simulink model "EHB_speedgoat_R2020a_V1"  (R2020a)
settings: Solver=FixedStepDiscrete  StartTime=0.0  StopTime=inf  FixedStep=0.001  RelTol=1e-3  EnableMultiTasking=on
model workspace (MAT data in the model file):
  A = Simulink.Signal
  A.DataType = 'uint8'
  A.Dimensions = 13
  A.DimensionsMode = 'auto'
  A.Complexity = 'auto'
  A.SampleTime = -1
  A.SamplingMode = 'auto'
  B = Simulink.Signal
  B.DataType = 'uint8'
  B.Dimensions = 13
  B.DimensionsMode = 'auto'
  B.Complexity = 'auto'
  B.SampleTime = -1
  B.SamplingMode = 'auto'
  C = Simulink.Signal
  C.DataType = 'uint8'
  C.Dimensions = 13
  C.DimensionsMode = 'auto'
  C.Complexity = 'auto'
  C.SampleTime = -1
  C.SamplingMode = 'auto'
  D = Simulink.Signal
  D.DataType = 'uint8'
  D.Dimensions = 13
  D.DimensionsMode = 'auto'
  D.Complexity = 'auto'
  D.SampleTime = -1
  D.SamplingMode = 'auto'
  E = Simulink.Signal
  E.DataType = 'uint8'
  E.Dimensions = 13
  E.DimensionsMode = 'auto'
  E.Complexity = 'auto'
  E.SampleTime = -1
  E.SamplingMode = 'auto'
  calin = [-9.96 -7.98 -5.98 -3.99 -1.994 0 1.995 3.992 5.99 7.98 9.97]
  calout = [-10 -8 -6 -4 -2 0 2 4 6 8 10]
undefined symbols (not defined in the file): Com1, none, ts_IO612
libraries: simulink x1436, xpcethercatlib x1223, yisutbxlib_utilities x256, xpcutilitieslib x156, hdlsllib x145, canmsglib x46, speedgoatlib_IO602_4 x11, speedgoatlib_IO611 x7, slrttcplib x4, CanManageLib x3, slrtlib x3, xpcseriallib x2
(part 1 of 30)
settings Model: xpc_rtwmakecfg_data=_xpcethercatlib_  SimulationMode=external  Creator=xiaoming  LastModifiedBy=17802
settings SolverCC: ConcurrentTasks=on  AutoInsertRateTranBlk=on
settings DataIOCC: SaveFormat=StructureWithTime  SaveState=on  SignalLoggingName=logsOut
settings OptimizationCC: BlockReduction=off  BooleanDataType=off  OptimizeBlockIOStorage=off  BufferReuse=off  GlobalBufferReuse=off  ExpressionFolding=off  LocalBlockOutputs=off  InitFltsAndDblsToZero=on  OptimizeDataStoreBuffers=off  BusAssignmentInplaceUpdate=off
settings DebuggingCC: SaveWithParameterizedLinksMsg=none  UnderspecifiedInitializationDetection=Classic  MergeDetectMultiDrivingBlocksExec=none  CheckExecutionContextPreStartOutputMsg=on  CheckExecutionContextRuntimeOutputMsg=on  SignalResolutionControl=TryResolveAllWithWarning  SFUnexpectedBacktrackingDiag=warning  SFNoUnconditionalDefaultTransitionDiag=warning  SFExecutionAtInitializationDiag=none  ArithmeticOperatorsInVariantConditions=warning
settings HardwareCC: ProdBitPerPointer=32  ProdBitPerSizeT=32  ProdBitPerPtrDiffT=32  ProdLargestAtomicFloat=None  ProdWordSize=32  ProdLongLongMode=on  ProdHWDeviceType=Generic->32-bit x86 compatible
settings ModelReferenceCC: PropagateSignalLabelsOutOfModel=off
settings SFSimCC: SimUseLocalCustomCode=off
settings RTWCC: Description=Simulink Real-Time  SystemTargetFile=slrt.tlc  TemplateMakefile=slrt_default_tmf  RTWUseLocalCustomCode=off  CodeExecutionProfiling=on  RTWCompilerOptimization=on
settings CodeAppCC: StateflowObjectComments=on
settings SimulinkRealTimeCC: SupportVariableSizeSignals=on  RL32LogTETModifier=off  xPCConcurrentTasks=on
settings ConfigComp: CovMetricSettings=dw  CovHtmlReporting=on  CovSaveCumulativeToWorkspaceVar=on  CovSaveSingleToWorkspaceVar=on  CovExternalEMLEnable=off  CovSFcnEnable=off

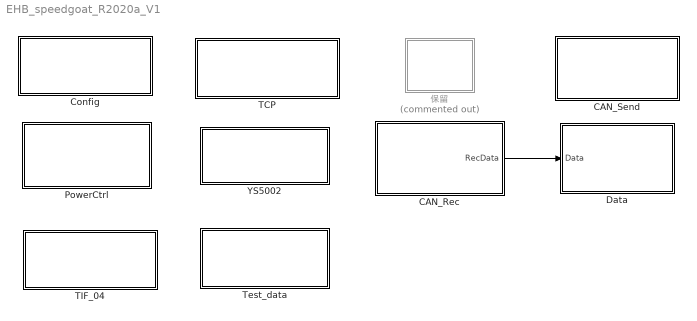
== system EHB_speedgoat_R2020a_V1 ==
  CAN_Rec : Subsystem
  CAN_Send : Subsystem
  Config : Subsystem
  Data : Subsystem
  PowerCtrl : Subsystem
  TCP : Subsystem
  TIF_04 : Subsystem
  Test_data : Subsystem
  YS5002 : Subsystem
  保留 : Subsystem  Commented=on
  wires:
  CAN_Rec/1(RecData) -> Data/1(Data)

== system EHB_speedgoat_R2020a_V1/CAN_Rec ==
  CAN Receive : Subsystem  TreatAsAtomicUnit=on
  RecData : Outport
  wires:
  CAN Receive/1(RecData) -> RecData/1

== system EHB_speedgoat_R2020a_V1/CAN_Send ==
  Bus Creator : BusCreator  Inputs=2
  CAN Transmit : Subsystem  TreatAsAtomicUnit=on
  Enable : BusSelector  OutputSignals=Trigger.Enable_CanTransmit
  Signal : Subsystem
  Trigger : Subsystem
  wires:
  Trigger/1(Trigger) -> Bus Creator/1  "Trigger"
  Signal/1(Signal) -> Bus Creator/2  "Signal"
  Bus Creator/1 -> CAN Transmit/1(Data), Enable/1  "Data"
  Enable/1 -> CAN Transmit/Enable  "<Enable_CanTransmit>"

== system EHB_speedgoat_R2020a_V1/Config ==
  CAN & LIN Setup : speedgoatlib_IO611/Legacy/CAN & LIN Setup  Commented=on  id=1  drvLtr=C:  PCISlot=-1  port1=CAN (HS/LS)  port2=CAN (HS/LS)  port3=LIN  port4=LIN  opModeCAN1=Highspeed (HS)  bdrCAN1=1 MBaud  usrBdrCAN1=[5, 1, 13, 2]  bdrFD1=5 MBaud  usrBdrFD1=[2, 1, 5, 2, 75, 5000]  stdAccMaskCAN1=[0, 0]  extAccMaskCAN1=[0, 0]  opModeCAN2=Highspeed (HS)  bdrCAN2=1 MBaud  usrBdrCAN2=[5, 1, 13, 2]  bdrFD2=5 MBaud  usrBdrFD2=[2, 1, 5, 2, 75, 5000]  stdAccMaskCAN2=[0, 0]  extAccMaskCAN2=[0, 0]  initStruct=[]  termStruct=[]  opModeLIN3=Master  bdrLIN3=19200  opModeLIN4=Slave  bdrLIN4=19200  protl=IO611  qtyMod=1  chNo=[1, 2, 3, 4]  ptTypes=[1, 1, 2, 2]  isProtlFD=[0, 0]  protlHelpIdx=[0, 1, 0, 1]  isFDMod=1
      settings: SourceProductName=Simulink Real-Time: Speedgoat I/O Blockset
  "CAN Setup " : speedgoatlib_IO602_4/Legacy/CAN Setup   moduletype=IO602  id=1  pciSlot=-1  chn1=CAN (HS)  chn2=CAN (HS)  chn3=CAN (HS)  chn4=CAN (HS)  initStruct=[]  termStruct=[]  ArbitrationbdrChn1=500 kBaud  ArbitrationManbdrChn1=[2,16,63,16]  FdbdrChn1=5.0 MBaud  FdManbdrChn1=[2,2,5,2]  ArbitrationbdrChn2=500 kBaud  ArbitrationManbdrChn2=[2,16,63,16]  FdbdrChn2=5.0 MBaud  FdManbdrChn2=[2,2,5,2]  ArbitrationbdrChn3=500 kBaud  ArbitrationManbdrChn3=[2,16,63,16]  FdbdrChn3=5.0 MBaud  FdManbdrChn3=[2,2,5,2]  ArbitrationbdrChn4=500 kBaud  ArbitrationManbdrChn4=[2,16,63,16]  FdbdrChn4=5.0 MBaud  FdManbdrChn4=[2,2,5,2]  moduleInitValues=[602 1 -1 -1]
      settings: SourceProductName=Simulink Real-Time: Speedgoat I/O Blockset
  Constant : Constant
  Gain{,1..5} (6 alike) : Gain
  HILReady : simulink/Logic and Bit Operations/Compare To Constant  relop===  const=8  OutDataTypeStr=boolean
  Selector : Selector  InputPortWidth=6  IndexOptions=Index vector (dialog)  Indices=[2]  OutputSizes=1
  TCP Client Configure : Subsystem  Priority=-1  AncestorBlock=slrttcplib/TCP Client Configure  InitFcn=|  TreatAsAtomicUnit=on  mask(slrttcpclientconfig){useHostTargetConn=off, clientAddress=192.168.0.55, clientPort=25001, SubnetMask=255.255.255.0, Gateway=0.0.0.0, remoteAddress=192.168.0.178, remotePort=4001, PciBus=[6], PciSlot=[0], PciFunction=[0]}
      | % Validate model
      | tcpvalidatemodel(gcb);
      mask prompts: useHostTargetConn "Use host-target connection"; clientAddress "Client IP address:"; clientPort "Client local port:"; SubnetMask "Subnet mask:"; remoteAddress "Remote server IP address:"; remotePort "Remote server port:"; PciBus "PCI Bus:"; PciSlot "Slot:"; PciFunction "Function:"
      mask help: Configure a TCP client application that uses the specified Ethernet interface.
      mask init:
      | % Validate mask parameter values
      | tcpslgate('privateTCPClientConfig', gcb, 'validateParams', clientAddress, clientPort, remoteAddress, remotePort, SubnetMask, Gateway, PciBus, PciSlot, PciFunction);
      mask Help: eval('xpcdoc(''TCP_ClientConfig'')');
      mask TypeOptions useHostTargetConn: TCP Client/useHostTargetConn | IP Configure/disable
      mask Callback useHostTargetConn: tcpslgate('privateTCPClientConfig', gcb, 'toggleMaskVisible');
      mask TypeOptions clientAddress: IP Configure/IpAddress | TCP Client/clientAddress
      mask TypeOptions clientPort: TCP Client/clientPort
      mask TypeOptions SubnetMask: IP Configure/SubnetMask
      mask TypeOptions Gateway: IP Configure/Gateway
      mask TypeOptions remoteAddress: TCP Client/remoteAddress
      mask TypeOptions remotePort: TCP Client/remotePort
      mask TypeOptions PciBus: IP Configure/PciBus
      mask TypeOptions PciSlot: IP Configure/PciSlot
      mask TypeOptions PciFunction: IP Configure/PciFunction
      mask DialogControl DescGroupVar Prompt: Configure TCP Client
      mask Display:
      | maskDisplay = tcpslgate('privateTCPClientConfig', gcb, 'dispStr', clientAddress, clientPort, remoteAddress, remotePort, SubnetMask, Gateway, PciBus, PciSlot, PciFunction);
      | disp(maskDisplay);
      | 
      | port_label('input', 1, 'Enable')
      | port_label('output', 1, 'Status')
  Terminator{,1..5} (6 alike) : Terminator
  YISU Toolbox Init : Subsystem  mask(ystbx_init){eniFile=D:\Matlab\EHB_Prj\data\ENI\HuDa.xml, deviceIdx=0, pciBus=7, pciSlot=0, pciFcn=0, outStatusInfo=on}
      mask prompts: eniFile "Config File(ENI):"; deviceIdx "Device Index:"; pciBus "PCI Bus:"; pciSlot "PCI Slot:"; pciFcn "PCI Function:"; outStatusInfo "Enable Status Info Output"
      mask help: 基于EtherCat Init模块，配置ENI文件并设定设备ID等信息
      mask DialogControl selectFile Prompt: Browse
      mask DialogControl selectFile Callback: ystbx.mask.callbacks.init_selectFile();
      mask DialogControl applyButton Prompt: Apply Modification
      mask DialogControl applyButton Callback: ystbx.mask.callbacks.maskApply();
      mask Display: disp('YISU Toolbox Init\nNetwork Device 0');port_label('output', 1, 'Status');
  wires:
  HILReady/1 -> Gain/1
  Selector/1 -> HILReady/1
  Constant/1 -> TCP Client Configure/5(In5), TCP Client Configure/4(In4), TCP Client Configure/3(In3), TCP Client Configure/2(In2), TCP Client Configure/1(In1)
  TCP Client Configure/1(Out1) -> Gain1/1
  TCP Client Configure/2(Out2) -> Gain2/1
  TCP Client Configure/3(Out3) -> Gain3/1
  TCP Client Configure/4(Out4) -> Gain4/1
  TCP Client Configure/5(Out5) -> Gain5/1
  YISU Toolbox Init/1(Status) -> Selector/1
  Gain/1 -> Terminator/1
  Gain1/1 -> Terminator1/1
  Gain2/1 -> Terminator2/1
  Gain3/1 -> Terminator3/1
  Gain4/1 -> Terminator4/1
  Gain5/1 -> Terminator5/1

== system EHB_speedgoat_R2020a_V1/Data ==
  note: EHB工作状态
  note: 制动状态反馈
  note: EHB故障等级
  note: 当前实际制动液压力
  note: 制动指令异常
  note: EHB液压力跟随轻微异常
  note: EHB液压力轻微震荡
  note: 温度传感器部分故障
  note: 温度传感器完全故障
  note: 液压力传感器故障
  note: 控制器温度过高
  note: 供电电压过低异常
  note: 供电电压过高异常
  note: EHB液压力跟随严重异常
  note: EHB液压力严重震荡
  note: 负载失配故障
  note: CAN通信故障
  note: EHB过流故障
  note: 电流传感器故障
  note: 供电电压过低故障
  note: 供电电压过高故障
  note: 功率开关故障
  note: 预驱故障
  note: EHB电机位置失效
  note: EHB软件版本号
  note: EHB硬件版本号
  note: 左前轮轮速
  note: 左前轮轮速有效性
  note: 右前轮轮速
  note: 右前轮轮速有效性
  note: 左后轮轮速
  note: 左后轮轮速有效性
  note: 右后轮轮速
  note: 右后轮轮速有效性
  Data : Inport
  Bus Selector : BusSelector  OutputSignals=CAN_Msg_0x125.EHB_Status,CAN_Msg_0x125.EHB_BrakeCondition,CAN_Msg_0x125.EHB_EHBFaultLevel,CAN_Msg_0x125.EHB_ActualPressure
  Bus Selector1 : BusSelector  OutputSignals=CAN_Msg_0x126.EHB_BrkReqWarn,CAN_Msg_0x126.EHB_PFolwFltLv1,CAN_Msg_0x126.EHB_PCtrlVibLv1,CAN_Msg_0x126.EHB_NTCFltLv1,CAN_Msg_0x126.EHB_NTCFltLv2,CAN_Msg_0x126.EHB_PSnsrFlt,CAN_Msg_0x126.EHB_OverTempWarn,CAN_Msg_0x126.EHB_USplyLowLv1,CAN_Msg_0x126.EHB_USplyHighLv1,CAN_Msg_0x126.EHB_PFolwFltLv2,CAN_Msg_0x126.EHB_PCtrlVibLv2,CAN_Msg_0x126.EHB_LoadMismatchFlt,CAN_Msg_0x126.EHB_CANBusOff,CAN_Msg_0x126.EHB_OverIFlt,CAN_Msg_0x126.EHB_ISnsrFlt,CAN_Msg_0x126.EHB_USplyLowLv2,CAN_Msg_0x126.EHB_USplyHighLv2,CAN_Msg_0x126.EHB_PwrSwtFlt,CAN_Msg_0x126.EHB_PwrDrvrFlt,CAN_Msg_0x126.EHB_MotPosnFlt,CAN_Msg_0x126.EHB_SoftwareVersion,CAN_Msg_0x126.EHB_HardwareVersion
  Bus Selector2 : BusSelector  OutputSignals=CAN_Msg_0x127.EHB_WhlFLSpd,CAN_Msg_0x127.EHB_WhlFLSpdVld,CAN_Msg_0x127.EHB_WhlFRSpd,CAN_Msg_0x127.EHB_WhlFRSpdVld,CAN_Msg_0x127.EHB_WhlRLSpd,CAN_Msg_0x127.EHB_WhlRLSpdVld,CAN_Msg_0x127.EHB_WhlRRSpd,CAN_Msg_0x127.EHB_WhlRRSpdVld
  Bus Selector3 : BusSelector  OutputSignals=Message_1_0x281.U_Current,Message_1_0x281.V_Current,Message_1_0x281.W_Current,Message_1_0x281.Angle1
  Bus Selector4 : BusSelector  OutputSignals=Message_3_0x283.ia_act,Message_3_0x283.ib_act
  Gain{,1..39} (40 alike) : Gain
  Terminator{,1..39} (40 alike) : Terminator
  wires:
  Data/1 -> Bus Selector3/1, Bus Selector2/1, [Data], Bus Selector1/1, Bus Selector/1
  Gain/1 -> Terminator/1
  Bus Selector/1 -> Gain/1  "<EHB_Status>"
  Gain1/1 -> Terminator1/1
  Bus Selector/2 -> Gain1/1  "<EHB_BrakeCondition>"
  Gain2/1 -> Terminator2/1
  Bus Selector/3 -> Gain2/1  "<EHB_EHBFaultLevel>"
  Gain3/1 -> Terminator3/1
  Bus Selector/4 -> Gain3/1  "<EHB_ActualPressure>"
  Gain7/1 -> Terminator7/1
  Gain6/1 -> Terminator6/1
  Gain5/1 -> Terminator5/1
  Gain4/1 -> Terminator4/1
  Bus Selector1/1 -> Gain4/1  "<EHB_BrkReqWarn>"
  Bus Selector1/2 -> Gain5/1  "<EHB_PFolwFltLv1>"
  Bus Selector1/3 -> Gain6/1  "<EHB_PCtrlVibLv1>"
  Bus Selector1/4 -> Gain7/1  "<EHB_NTCFltLv1>"
  Gain8/1 -> Terminator8/1
  Gain9/1 -> Terminator9/1
  Gain10/1 -> Terminator10/1
  Gain11/1 -> Terminator11/1
  Gain13/1 -> Terminator13/1
  Gain12/1 -> Terminator12/1
  Gain19/1 -> Terminator19/1
  Gain18/1 -> Terminator18/1
  Gain14/1 -> Terminator14/1
  Gain15/1 -> Terminator15/1
  Gain16/1 -> Terminator16/1
  Gain17/1 -> Terminator17/1
  Gain25/1 -> Terminator25/1
  Gain24/1 -> Terminator24/1
  Gain23/1 -> Terminator23/1
  Gain22/1 -> Terminator22/1
  Gain26/1 -> Terminator26/1
  Gain27/1 -> Terminator27/1
  Bus Selector1/5 -> Gain8/1  "<EHB_NTCFltLv2>"
  Bus Selector1/6 -> Gain9/1  "<EHB_PSnsrFlt>"
  Bus Selector1/7 -> Gain10/1  "<EHB_OverTempWarn>"
  Bus Selector1/8 -> Gain11/1  "<EHB_USplyLowLv1>"
  Bus Selector1/9 -> Gain14/1  "<EHB_USplyHighLv1>"
  Bus Selector1/10 -> Gain15/1  "<EHB_PFolwFltLv2>"
  Bus Selector1/11 -> Gain16/1  "<EHB_PCtrlVibLv2>"
  Bus Selector1/12 -> Gain17/1  "<EHB_LoadMismatchFlt>"
  Bus Selector1/13 -> Gain18/1  "<EHB_CANBusOff>"
  Bus Selector1/14 -> Gain19/1  "<EHB_OverIFlt>"
  Bus Selector1/15 -> Gain12/1  "<EHB_ISnsrFlt>"
  Bus Selector1/16 -> Gain13/1  "<EHB_USplyLowLv2>"
  Bus Selector1/17 -> Gain22/1  "<EHB_USplyHighLv2>"
  Bus Selector1/18 -> Gain23/1  "<EHB_PwrSwtFlt>"
  Bus Selector1/19 -> Gain24/1  "<EHB_PwrDrvrFlt>"
  Bus Selector1/20 -> Gain25/1  "<EHB_MotPosnFlt>"
  Bus Selector1/21 -> Gain26/1  "<EHB_SoftwareVersion>"
  Bus Selector1/22 -> Gain27/1  "<EHB_HardwareVersion>"
  Gain29/1 -> Terminator29/1
  Gain28/1 -> Terminator28/1
  Gain21/1 -> Terminator21/1
  Gain20/1 -> Terminator20/1
  Gain30/1 -> Terminator30/1
  Gain31/1 -> Terminator31/1
  Gain32/1 -> Terminator32/1
  Gain33/1 -> Terminator33/1
  Bus Selector2/1 -> Gain20/1  "<EHB_WhlFLSpd>"
  Bus Selector2/2 -> Gain21/1  "<EHB_WhlFLSpdVld>"
  Bus Selector2/3 -> Gain28/1  "<EHB_WhlFRSpd>"
  Bus Selector2/4 -> Gain29/1  "<EHB_WhlFRSpdVld>"
  Bus Selector2/5 -> Gain30/1  "<EHB_WhlRLSpd>"
  Bus Selector2/6 -> Gain31/1  "<EHB_WhlRLSpdVld>"
  Bus Selector2/7 -> Gain32/1  "<EHB_WhlRRSpd>"
  Bus Selector2/8 -> Gain33/1  "<EHB_WhlRRSpdVld>"
  Gain37/1 -> Terminator37/1
  Gain36/1 -> Terminator36/1
  Gain35/1 -> Terminator35/1
  Gain34/1 -> Terminator34/1
  Bus Selector3/1 -> Gain34/1  "<U_Current>"
  Bus Selector3/2 -> Gain35/1  "<V_Current>"
  Bus Selector3/3 -> Gain36/1  "<W_Current>"
  Bus Selector3/4 -> Gain37/1  "<Angle1>"
  [Data] -> Bus Selector4/1
  Gain38/1 -> Terminator38/1
  Gain39/1 -> Terminator39/1
  Bus Selector4/1 -> Gain38/1  "<ia_act>"
  Bus Selector4/2 -> Gain39/1  "<ib_act>"

== system EHB_speedgoat_R2020a_V1/PowerCtrl ==
  CurrSet[A] : Constant  OutDataTypeStr=uint16
  OnOff : Constant  OutDataTypeStr=uint8
  PowerCtrl : Subsystem
  PowerPosSet[W] : Constant  Value=6000  OutDataTypeStr=uint16
  Toggle Switch : ToggleSwitchBlock  LabelPosition=Hide
      settings: Values={{'Off', 'On'}, [0 1]}
  VoltValue[V] : Constant  Value=12  OutDataTypeStr=uint32
  wires:
  CurrSet[A]/1 -> PowerCtrl/3(CurrSet[A])  "CurrSet[A]"
  [Power_V] -> PowerCtrl/1(VoltValue[V])  "VoltValue[V]"
  OnOff/1 -> PowerCtrl/2(OnOff)  "OnOff"
  PowerPosSet[W]/1 -> PowerCtrl/4(PowerPosSet[W])  "PowerPosSet[W]"

== system EHB_speedgoat_R2020a_V1/TCP ==
  Constant{,1..3} (4 alike) : Constant
  Counter Limited1 : simulink/Sources/Counter Limited  uplimit=7  tsamp=0.1
  Counter Limited3 : simulink/Sources/Counter Limited  uplimit=6  tsamp=0.1
  From1 : From  Commented=on  GotoTag=YS4008_M_3  TagVisibility=global
  From11 : From  Commented=on  GotoTag=YS4008_M_2  TagVisibility=global
  From15 : From  Commented=on  GotoTag=YS7501_M  TagVisibility=global
  From18 : From  Commented=on  GotoTag=YS4008_M_4  TagVisibility=global
  From19 : From  Commented=on  GotoTag=YS4008_M_1  TagVisibility=global
  From20 : From  Commented=on  GotoTag=YS4008_M_5  TagVisibility=global
  From21 : From  Commented=on  GotoTag=YS4008_M_6  TagVisibility=global
  From22 : From  Commented=on  GotoTag=YS4020_M_2_1  TagVisibility=global
  From24 : From  Commented=on  GotoTag=YS4020_M_2_2  TagVisibility=global
  From6 : From  Commented=on  GotoTag=YS4020_M_1_2  TagVisibility=global
  From9 : From  Commented=on  GotoTag=YS4020_M_1_1  TagVisibility=global
  Ground{,1..10} (11 alike) : Ground
  Multiport Switch1 : MultiPortSwitch  DataPortOrder=Zero-based contiguous  Inputs=8  DiagnosticForDefault=None  zeroidx=on
  Multiport Switch2 : MultiPortSwitch  DataPortOrder=Zero-based contiguous  Inputs=7  DiagnosticForDefault=None  zeroidx=on
  TCP Send : slrttcplib/TCP Send  socketAddPortVal=Client: 192.168.0.55:25001  sampleTime=-1
      settings: SourceProductBaseCode=XP
  TCP Send1 : slrttcplib/TCP Send  socketAddPortVal=Client: 192.168.0.55:25002  sampleTime=-1
      settings: SourceProductBaseCode=XP
  TCP Send2 : slrttcplib/TCP Send  socketAddPortVal=Client: 192.168.0.55:25003  sampleTime=-1
      settings: SourceProductBaseCode=XP
  TCP Send3 : slrttcplib/TCP Send  socketAddPortVal=Client: 192.168.0.55:25004  sampleTime=-1
      settings: SourceProductBaseCode=XP
  Terminator{,1..3} (4 alike) : Terminator
  Width{,1..3} (4 alike) : Width
  wires:
  Width/1 -> TCP Send/3
  [PowerPosSet] -> Multiport Switch2/4
  [CurrSet] -> Multiport Switch2/3
  [VoltSet] -> Multiport Switch2/2
  Ground/1 -> Multiport Switch1/2
  Multiport Switch1/1 -> TCP Send/2, Width/1
  [YS5002] -> Multiport Switch2/5
  Ground8/1 -> Multiport Switch2/6
  Ground9/1 -> Multiport Switch2/7
  Ground4/1 -> Multiport Switch1/3
  Ground1/1 -> Multiport Switch1/4
  Ground5/1 -> Multiport Switch1/5
  [Enable] -> Width2/1, TCP Send2/2
  Ground6/1 -> Multiport Switch1/7
  Ground2/1 -> Multiport Switch1/6
  Ground10/1 -> Multiport Switch2/8
  Constant/1 -> TCP Send/1
  TCP Send/1 -> Terminator/1
  TCP Send1/1 -> Terminator1/1
  Constant1/1 -> TCP Send1/1
  Multiport Switch2/1 -> TCP Send1/2, Width1/1
  Width1/1 -> TCP Send1/3
  Constant2/1 -> TCP Send2/1
  Width2/1 -> TCP Send2/3
  TCP Send2/1 -> Terminator2/1
  Counter Limited1/1 -> Multiport Switch1/1
  Counter Limited3/1 -> Multiport Switch2/1
  TCP Send3/1 -> Terminator3/1
  Width3/1 -> TCP Send3/3
  Constant3/1 -> TCP Send3/1
  [CANOpenInit] -> TCP Send3/2, Width3/1
  Ground3/1 -> Multiport Switch1/8
  Ground7/1 -> Multiport Switch1/9

== system EHB_speedgoat_R2020a_V1/TIF_04 ==
  CB2020_1 : Subsystem
  CB2020_2 : Subsystem  Commented=on
  CB2020_3 : Subsystem

== system EHB_speedgoat_R2020a_V1/Test_data ==
  note: U相电流
  note: 点火信号（电压）
  note: 压力传感器（电压）
  note: 程控电源（电压）
  note: 5V（电压）
  note: V相电流
  note: W相电流
  12V_DAC_CH1 : Constant  Value=0  OutDataTypeStr=Inherit: Inherit via back propagation
  DAC_CH1 : Constant  Value=0  OutDataTypeStr=double
  Gain{1..4} (4 alike) : Gain
  Saturation : Saturate  UpperLimit=5  LowerLimit=0
  Terminator{1..4} (4 alike) : Terminator
  VoltValue[V] : Constant  Value=12  OutDataTypeStr=uint32
  tag scope: PowerOn_Off=global, Power_V=global, Pressure_V=global
  wires:
  Gain1/1 -> Terminator1/1
  Gain2/1 -> Terminator2/1
  Gain3/1 -> Terminator3/1
  Gain4/1 -> Terminator4/1
  12V_DAC_CH1/1 -> [PowerOn_Off]  "PowerOn_Off"
  DAC_CH1/1 -> Saturation/1  "Pressure_V"
  VoltValue[V]/1 -> [Power_V]  "Power_V"
  [Power_5V] -> Gain1/1  "Power_5V"
  [Current_U] -> Gain2/1  "Current_U"
  [Current_V] -> Gain3/1  "Current_V"
  [Current_W] -> Gain4/1  "Current_W"
  Saturation/1 -> [Pressure_V]

== system EHB_speedgoat_R2020a_V1/YS5002 ==
  Bitwise OR : simulink/Logic and Bit Operations/Bitwise Operator  logicop=OR  UseBitMask=off  BitMask=bin2dec('11011001')  BitMaskRealWorld=Stored Integer
  Bus Creator : BusCreator  Inputs=4
  Detect Change : simulink/Logic and Bit Operations/Detect Change  vinit=0  OutDataTypeStr=boolean
  Mux : Mux
  PS{1..4} (4 alike) : Constant  OutDataTypeStr=boolean
  YS5002_M_PowerCtrl : Subsystem
  tag scope: YS5002=global
  wires:
  PS1/1 -> Mux/1, Bus Creator/1  "PS1"
  PS2/1 -> Mux/2, Bus Creator/2  "PS2"
  PS3/1 -> Mux/3, Bus Creator/3  "PS3"
  Bus Creator/1 -> YS5002_M_PowerCtrl/1(YS5002_M)  "YS5002_M"
  PS4/1 -> Mux/4, Bus Creator/4  "PS4"
  YS5002_M_PowerCtrl/1(Output) -> [YS5002]
  Mux/1 -> Detect Change/1
  Detect Change/1 -> Bitwise OR/1
  Bitwise OR/1 -> YS5002_M_PowerCtrl/Enable

== system EHB_speedgoat_R2020a_V1/保留 ==
  IO602 : Subsystem  Commented=on
  IO611 : Subsystem  Commented=on
  RS232 : Subsystem  Commented=on
  TIF_01 : Subsystem  Commented=on
  TIF_02 : Subsystem  Commented=on
  TIF_03 : Subsystem  Commented=on
  TIF_06 : Subsystem  Commented=on
  YS4008 : Subsystem  Commented=on
  YS7501_M : Subsystem  Commented=on

== system EHB_speedgoat_R2020a_V1/CAN_Rec/CAN Receive ==
  Bus Creator : BusCreator  Inputs=10
  CAN Read : speedgoatlib_IO602_4/Legacy/CAN Read  id=1  ts=-1  channel=1  messageType=CAN  canType=CAN (HS)  BusOutput=on  initValues=[602 1 -1 0 1 1 1]
      settings: SourceProductName=Simulink Real-Time: Speedgoat I/O Blockset
  CAN_Msg_0x125 : Subsystem  TreatAsAtomicUnit=on
  CAN_Msg_0x126 : Subsystem  TreatAsAtomicUnit=on
  CAN_Msg_0x127 : Subsystem  TreatAsAtomicUnit=on
  Debug1_0x287 : Subsystem  TreatAsAtomicUnit=on
  Debug_0x286 : Subsystem  TreatAsAtomicUnit=on
  Message_1_0x281 : Subsystem  TreatAsAtomicUnit=on
  Message_2_0x282 : Subsystem  TreatAsAtomicUnit=on
  Message_3_0x283 : Subsystem  TreatAsAtomicUnit=on
  Message_4_0x284 : Subsystem  TreatAsAtomicUnit=on
  Message_5_0x285 : Subsystem  TreatAsAtomicUnit=on
  RecMsgCheck{1..10} (10 alike) : Constant  OutDataTypeStr=boolean
  While Iterator : WhileIterator  MaxIters=500  WhileBlockType=do-while
  RecData : Outport
  wires:
  CAN Read/1 -> While Iterator/1
  CAN Read/2 -> [CANMsg]
  RecMsgCheck1/1 -> Debug_0x286/Enable
  [CANMsg] -> Debug_0x286/1(CAN Msg)
  Debug_0x286/1(Debug) -> [Debug_0x286]
  RecMsgCheck2/1 -> Debug1_0x287/Enable
  [CANMsg] -> Debug1_0x287/1(CAN Msg)
  Debug1_0x287/1(Debug1) -> [Debug1_0x287]
  RecMsgCheck3/1 -> Message_1_0x281/Enable
  [CANMsg] -> Message_1_0x281/1(CAN Msg)
  Message_1_0x281/1(Message_1) -> [Message_1_0x281]
  RecMsgCheck4/1 -> Message_2_0x282/Enable
  [CANMsg] -> Message_2_0x282/1(CAN Msg)
  Message_2_0x282/1(Message_2) -> [Message_2_0x282]
  RecMsgCheck5/1 -> Message_3_0x283/Enable
  [CANMsg] -> Message_3_0x283/1(CAN Msg)
  Message_3_0x283/1(Message_3) -> [Message_3_0x283]
  RecMsgCheck6/1 -> Message_4_0x284/Enable
  [CANMsg] -> Message_4_0x284/1(CAN Msg)
  Message_4_0x284/1(Message_4) -> [Message_4_0x284]
  RecMsgCheck7/1 -> Message_5_0x285/Enable
  [CANMsg] -> Message_5_0x285/1(CAN Msg)
  Message_5_0x285/1(Message_5) -> [Message_5_0x285]
  [Debug_0x286] -> Bus Creator/1  "Debug_0x286"
  [Debug1_0x287] -> Bus Creator/2  "Debug1_0x287"
  [Message_1_0x281] -> Bus Creator/3  "Message_1_0x281"
  [Message_2_0x282] -> Bus Creator/4  "Message_2_0x282"
  [Message_3_0x283] -> Bus Creator/5  "Message_3_0x283"
  [Message_4_0x284] -> Bus Creator/6  "Message_4_0x284"
  [Message_5_0x285] -> Bus Creator/7  "Message_5_0x285"
  Bus Creator/1 -> RecData/1  "RecData"
  CAN_Msg_0x125/1(CAN_Msg_0x125) -> [CAN_Msg_0x125]
  [CANMsg] -> CAN_Msg_0x125/1(CAN Msg)
  RecMsgCheck8/1 -> CAN_Msg_0x125/Enable
  RecMsgCheck9/1 -> CAN_Msg_0x126/Enable
  [CANMsg] -> CAN_Msg_0x126/1(CAN Msg)
  CAN_Msg_0x126/1(CAN_Msg_0x126) -> [CAN_Msg_0x126]
  RecMsgCheck10/1 -> CAN_Msg_0x127/Enable
  [CANMsg] -> CAN_Msg_0x127/1(CAN Msg)
  CAN_Msg_0x127/1(CAN_Msg_0x127) -> [CAN_Msg_0x127]
  [CAN_Msg_0x125] -> Bus Creator/8  "CAN_Msg_0x125"
  [CAN_Msg_0x126] -> Bus Creator/9  "CAN_Msg_0x126"
  [CAN_Msg_0x127] -> Bus Creator/10  "CAN_Msg_0x127"

== system EHB_speedgoat_R2020a_V1/CAN_Send/CAN Transmit ==
  Data : Inport
  Enable : EnablePort
  Data1 : BusSelector  OutputSignals=Trigger.VCU_Msg,Signal.VCU_Msg
  Enable1 : BusSelector  OutputSignals=Enable_VCU_Msg
  VCU_Msg : Subsystem  TreatAsAtomicUnit=on
  wires:
  Data/1 -> Data1/1
  Data1/1 -> VCU_Msg/1(Trigger), Enable1/1  "<VCU_Msg>"
  Data1/2 -> VCU_Msg/2(VCU_Msg)  "<VCU_Msg>"
  Enable1/1 -> VCU_Msg/Enable  "<Enable_VCU_Msg>"

== system EHB_speedgoat_R2020a_V1/CAN_Send/Signal ==
  Bus Creator : BusCreator  Inputs=1
  CAN_Msg_VCU : Subsystem
  Signal : Outport
  wires:
  CAN_Msg_VCU/1(VCU_Msg) -> Bus Creator/1  "VCU_Msg"
  Bus Creator/1 -> Signal/1  "Signal"

== system EHB_speedgoat_R2020a_V1/CAN_Send/Trigger ==
  Bus Creator : BusCreator  Inputs=2
  Enable_CanTransmit : Constant
  Trigger_VCU_Msg : Subsystem
  Trigger : Outport
  wires:
  Trigger_VCU_Msg/1(VCU_Msg) -> Bus Creator/1  "VCU_Msg"
  Enable_CanTransmit/1 -> Bus Creator/2  "Enable_CanTransmit"
  Bus Creator/1 -> Trigger/1  "Trigger"

== system EHB_speedgoat_R2020a_V1/Config/TCP Client Configure ==
  In1 : Inport
  In2 : Inport  Port=2
  In3 : Inport  Port=3
  In4 : Inport  Port=4
  In5 : Inport  Port=5
  IP Configure : S-Function  Priority=-2  InitFcn=|  FunctionName=slrtIPConfig  Parameters=ipAdd, snMask, gwAdd, gwDest, 0, '', '', PciBus, PciSlot, PciFunction, tune, disable  SFunctionDeploymentMode=off  EnableBusSupport=off  mask(slrtudpconfigure){IpAddress=192.168.0.55, SubnetMask=255.255.255.0, Gateway=0.0.0.0, PciBus=PciBus, PciSlot=PciSlot, PciFunction=PciFunction, ID=1, tune=0, disable=off}
      | % Validate model
      | udpvalidatemodel(gcb);
      mask prompts: IpAddress "Local IP address:"; SubnetMask "Subnet mask:"; PciBus "PCI Bus:"; PciSlot "Slot:"; PciFunction "Function:"; ID "deviceID:"
      mask help: Initialize Ethernet network interface to use for IP communication in real-time applications.
      mask init:
      | % Validate mask parameter values
      | [ipAdd, snMask, gwAdd, gwDest] = ...
      |     udpslgate('privateIPConfigure', 'validateParams', IpAddress,...
      |     PciBus, PciSlot, PciFunction, SubnetMask, Gateway,...
      |     0,... % enableMulticast
      |     '',...% Multicast address
      |     '',...% Multicast mask
      |     disable);
      mask Help: eval('xpcdoc(''IP_Config'')');
      mask DialogControl DescGroupVar Prompt: IP Configure
      mask Display:
      | maskDisplay = 'Configure IP';
      | disp(maskDisplay)
      | 
      | if tune
      |     port_label('output', 1, 'Curr Free')
      |     port_label('output', 2, 'High Free')
      |     port_label('output', 3, 'Low Free')
      | end
  TCP Client : S-Function  Priority=-1  InitFcn=|  FunctionName=slrtTCPClient  Parameters=clientAdd, clientPort, remoteAdd, remotePort, useHostTargetComm  SFunctionDeploymentMode=off  EnableBusSupport=off  mask(slrttcpclient){useHostTargetConn=off, clientAddress=192.168.0.55, clientPort=clientPort, remoteAddress=192.168.0.178, remotePort=remotePort}
      | % Validate model
      | tcpvalidatemodel(gcb);
      mask prompts: useHostTargetConn "Use host-target connection"; clientAddress "Client IP address:"; clientPort "Client local port:"; remoteAddress "Remote server IP address:"; remotePort "Remote server port:"
      mask help: Configure TCP Client
      mask init:
      | % Validate mask parameter values
      | [clientAdd, remoteAdd, useHostTargetComm] = ...
      |     tcpslgate('privateTCPClient', 'validateParams', gcb, clientAddress, clientPort, remoteAddress, remotePort);
      mask Help: eval('xpcdoc(''TCP_Client'')');
      mask Callback useHostTargetConn: tcpslgate('privateTCPClient', 'toggleMaskVisible', gcb);
      mask Callback clientAddress: %udpslgate('privateupdateIPlist', gcb, 'UpdateIPList');
      mask DialogControl DescGroupVar Prompt: TCP Client
      mask Display:
      | maskDisplay = tcpslgate('privateTCPClient', 'dispStr', gcb, clientAddress, clientPort, remoteAddress, remotePort);
      | disp(maskDisplay);
      | 
      | port_label('input', 1, 'Connect')
      | port_label('output', 1, 'Status')
  TCP Client1 : S-Function  Priority=-1  InitFcn=|  FunctionName=slrtTCPClient  Parameters=clientAdd, clientPort, remoteAdd, remotePort, useHostTargetComm  SFunctionDeploymentMode=off  EnableBusSupport=off  mask(slrttcpclient){useHostTargetConn=off, clientAddress=192.168.0.55, clientPort=25002, remoteAddress=192.168.0.178, remotePort=4001}
      | % Validate model
      | tcpvalidatemodel(gcb);
      mask prompts: useHostTargetConn "Use host-target connection"; clientAddress "Client IP address:"; clientPort "Client local port:"; remoteAddress "Remote server IP address:"; remotePort "Remote server port:"
      mask help: Configure TCP Client
      mask init:
      | % Validate mask parameter values
      | [clientAdd, remoteAdd, useHostTargetComm] = ...
      |     tcpslgate('privateTCPClient', 'validateParams', gcb, clientAddress, clientPort, remoteAddress, remotePort);
      mask Help: eval('xpcdoc(''TCP_Client'')');
      mask Callback useHostTargetConn: tcpslgate('privateTCPClient', 'toggleMaskVisible', gcb);
      mask Callback clientAddress: %udpslgate('privateupdateIPlist', gcb, 'UpdateIPList');
      mask DialogControl DescGroupVar Prompt: TCP Client
      mask Display:
      | maskDisplay = tcpslgate('privateTCPClient', 'dispStr', gcb, clientAddress, clientPort, remoteAddress, remotePort);
      | disp(maskDisplay);
      | 
      | port_label('input', 1, 'Connect')
      | port_label('output', 1, 'Status')
  TCP Client2 : S-Function  Priority=-1  InitFcn=|  FunctionName=slrtTCPClient  Parameters=clientAdd, clientPort, remoteAdd, remotePort, useHostTargetComm  SFunctionDeploymentMode=off  EnableBusSupport=off  mask(slrttcpclient){useHostTargetConn=off, clientAddress=192.168.0.55, clientPort=25003, remoteAddress=192.168.0.178, remotePort=4001}
      | % Validate model
      | tcpvalidatemodel(gcb);
      mask prompts: useHostTargetConn "Use host-target connection"; clientAddress "Client IP address:"; clientPort "Client local port:"; remoteAddress "Remote server IP address:"; remotePort "Remote server port:"
      mask help: Configure TCP Client
      mask init:
      | % Validate mask parameter values
      | [clientAdd, remoteAdd, useHostTargetComm] = ...
      |     tcpslgate('privateTCPClient', 'validateParams', gcb, clientAddress, clientPort, remoteAddress, remotePort);
      mask Help: eval('xpcdoc(''TCP_Client'')');
      mask Callback useHostTargetConn: tcpslgate('privateTCPClient', 'toggleMaskVisible', gcb);
      mask Callback clientAddress: %udpslgate('privateupdateIPlist', gcb, 'UpdateIPList');
      mask DialogControl DescGroupVar Prompt: TCP Client
      mask Display:
      | maskDisplay = tcpslgate('privateTCPClient', 'dispStr', gcb, clientAddress, clientPort, remoteAddress, remotePort);
      | disp(maskDisplay);
      | 
      | port_label('input', 1, 'Connect')
      | port_label('output', 1, 'Status')
  TCP Client3 : S-Function  Priority=-1  InitFcn=|  FunctionName=slrtTCPClient  Parameters=clientAdd, clientPort, remoteAdd, remotePort, useHostTargetComm  SFunctionDeploymentMode=off  EnableBusSupport=off  mask(slrttcpclient){useHostTargetConn=off, clientAddress=192.168.0.55, clientPort=25004, remoteAddress=192.168.0.178, remotePort=4001}
      | % Validate model
      | tcpvalidatemodel(gcb);
      mask prompts: useHostTargetConn "Use host-target connection"; clientAddress "Client IP address:"; clientPort "Client local port:"; remoteAddress "Remote server IP address:"; remotePort "Remote server port:"
      mask help: Configure TCP Client
      mask init:
      | % Validate mask parameter values
      | [clientAdd, remoteAdd, useHostTargetComm] = ...
      |     tcpslgate('privateTCPClient', 'validateParams', gcb, clientAddress, clientPort, remoteAddress, remotePort);
      mask Help: eval('xpcdoc(''TCP_Client'')');
      mask Callback useHostTargetConn: tcpslgate('privateTCPClient', 'toggleMaskVisible', gcb);
      mask Callback clientAddress: %udpslgate('privateupdateIPlist', gcb, 'UpdateIPList');
      mask DialogControl DescGroupVar Prompt: TCP Client
      mask Display:
      | maskDisplay = tcpslgate('privateTCPClient', 'dispStr', gcb, clientAddress, clientPort, remoteAddress, remotePort);
      | disp(maskDisplay);
      | 
      | port_label('input', 1, 'Connect')
      | port_label('output', 1, 'Status')
  TCP Client4 : S-Function  Priority=-1  InitFcn=|  FunctionName=slrtTCPClient  Parameters=clientAdd, clientPort, remoteAdd, remotePort, useHostTargetComm  SFunctionDeploymentMode=off  EnableBusSupport=off  mask(slrttcpclient){useHostTargetConn=off, clientAddress=192.168.0.55, clientPort=25005, remoteAddress=192.168.0.178, remotePort=4001}
      | % Validate model
      | tcpvalidatemodel(gcb);
      mask prompts: useHostTargetConn "Use host-target connection"; clientAddress "Client IP address:"; clientPort "Client local port:"; remoteAddress "Remote server IP address:"; remotePort "Remote server port:"
      mask help: Configure TCP Client
      mask init:
      | % Validate mask parameter values
      | [clientAdd, remoteAdd, useHostTargetComm] = ...
      |     tcpslgate('privateTCPClient', 'validateParams', gcb, clientAddress, clientPort, remoteAddress, remotePort);
      mask Help: eval('xpcdoc(''TCP_Client'')');
      mask Callback useHostTargetConn: tcpslgate('privateTCPClient', 'toggleMaskVisible', gcb);
      mask Callback clientAddress: %udpslgate('privateupdateIPlist', gcb, 'UpdateIPList');
      mask DialogControl DescGroupVar Prompt: TCP Client
      mask Display:
      | maskDisplay = tcpslgate('privateTCPClient', 'dispStr', gcb, clientAddress, clientPort, remoteAddress, remotePort);
      | disp(maskDisplay);
      | 
      | port_label('input', 1, 'Connect')
      | port_label('output', 1, 'Status')
  Out1 : Outport  VectorParamsAs1DForOutWhenUnconnected=off
  Out2 : Outport  Port=2  VectorParamsAs1DForOutWhenUnconnected=off
  Out3 : Outport  Port=3  VectorParamsAs1DForOutWhenUnconnected=off
  Out4 : Outport  Port=4  VectorParamsAs1DForOutWhenUnconnected=off
  Out5 : Outport  Port=5  VectorParamsAs1DForOutWhenUnconnected=off
  wires:
  TCP Client/1 -> Out1/1
  In1/1 -> TCP Client/1
  In2/1 -> TCP Client1/1
  TCP Client1/1 -> Out2/1
  TCP Client2/1 -> Out3/1
  In3/1 -> TCP Client2/1
  In4/1 -> TCP Client3/1
  TCP Client3/1 -> Out4/1
  TCP Client4/1 -> Out5/1
  In5/1 -> TCP Client4/1

== system EHB_speedgoat_R2020a_V1/Config/YISU Toolbox Init ==
  EtherCAT Init : xpcethercatlib/EtherCAT Init   Priority=0  config_file=D:\Matlab\EHB_Prj\data\ENI\HuDa.xml  device_id=0  pci_bus=7  pci_slot=0  pci_function=0  initstate=2  dctuning=0  enaDebug=off  enaDC=on  errLink=off  masterDbg=off  stateChgDbg=off  baseClock=off  masterCfg=off  logFile='c:\dbglog.txt'  sample_time=0.001000  DCMode=0
      settings: SourceProductBaseCode=XP
  Status : Outport
  wires:
  EtherCAT Init/1 -> Status/1

== system EHB_speedgoat_R2020a_V1/PowerCtrl/PowerCtrl ==
  VoltValue[V] : Inport
  OnOff : Inport  Port=2
  CurrSet[A] : Inport  Port=3
  PowerPosSet[W] : Inport  Port=4
  CANOpenInit1 : Subsystem
  CurrSet1 : Subsystem
  Enable1 : Subsystem
  IT_M3902D_Ctrl_Trigger : Subsystem
  PowerPosSet1 : Subsystem
  Start : Constant  OutDataTypeStr=boolean
  VoltSet1 : Subsystem
  tag scope: CANOpenInit=global, CurrSet=global, Enable=global, PowerPosSet=global, VoltSet=global
  wires:
  Start/1 -> CANOpenInit1/1(Start/Stop)
  VoltValue[V]/1 -> VoltSet1/1(VoltValue[V]), IT_M3902D_Ctrl_Trigger/1(VoltValue)
  OnOff/1 -> Enable1/1(OnOff), IT_M3902D_Ctrl_Trigger/2(OnOff)
  PowerPosSet[W]/1 -> PowerPosSet1/1(PowerPosSet[W]), IT_M3902D_Ctrl_Trigger/4(PowerPosSet)
  CurrSet[A]/1 -> CurrSet1/1(CurrSet[A]), IT_M3902D_Ctrl_Trigger/3(CurrSet)
  IT_M3902D_Ctrl_Trigger/1(HVRealy_Ctrl_Trigger) -> PowerPosSet1/Trigger, CurrSet1/Trigger, Enable1/Trigger, VoltSet1/Trigger  "Trigger"
  CANOpenInit1/1(Output) -> [CANOpenInit]
  VoltSet1/1(Output) -> [VoltSet]
  Enable1/1(Output) -> [Enable]
  CurrSet1/1(Output) -> [CurrSet]
  PowerPosSet1/1(Output) -> [PowerPosSet]

== system EHB_speedgoat_R2020a_V1/TIF_04/CB2020_1 ==
  ADC : Subsystem  mask(simucat_adc){deviceID=0, boxNum=Box 5 (Analog Board), channel1=on, channel2=on, channel3=on, channel4=off, channel5=off, channel6=off, channel7=off, channel8=off, channel9=off, channel10=off, channel11=off, channel12=off, channel13=off, channel14=off, channel15=off, channel16=off}
      mask prompts: deviceID "Device Index:"; boxNum "Select a box:"; channel1 "1"; channel2 "2"; channel3 "3"; channel4 "4"; channel5 "5"; channel6 "6"; channel7 "7"; channel8 "8"; channel9 "9"; channel10 "10"; channel11 "11"; channel12 "12"; channel13 "13"; channel14 "14"; channel15 "15"; channel16 "16"
      mask help:
      | SimuCat系列模拟板卡驱动模块。
      | 功能：模拟量转换数字量。通道数：16
      mask TypeOptions deviceID: 0 | 1 | 2 | 3 | 4 | 5 | 6 | 7 | 8 | 9 | 10 | 11 | 12 | 13 | 14 | 15
      mask TypeOptions boxNum: Box 5 (Analog Board) | Box 6 (Analog Board) | Box 7 (Analog Board)
      mask DialogControl refreshButton Prompt: Refresh
      mask DialogControl refreshButton Callback: ystbx.mask.callbacks.refreshBoxList
      mask DialogControl selectChannel Prompt: Select channels:
      mask DialogControl Dummy Prompt: (Add text here)
      mask DialogControl channelSelectAll Prompt: Select All
      mask DialogControl channelSelectAll Callback: ystbx.mask.callbacks.selectAllChannels();
      mask DialogControl channelClearAll Prompt: Clear All
      mask DialogControl channelClearAll Callback: ystbx.mask.callbacks.clearAllChannels();
      mask DialogControl applyButton Prompt: Apply Modification
      mask DialogControl applyButton Callback: ystbx.mask.callbacks.maskApply();
      mask Display: disp('CB2020(Analog Board)\nanalog-to-digital converter\nNetwork Device 0\nBox 5 (Analog Board)');port_label('output',1,'ADC_CH1[V]');port_label('output',2,'ADC_CH2[V]');port_label('output',3,'ADC_CH3[V]');
  AI1 : Subsystem
  AI2 : Subsystem
  AI3 : Subsystem
  DAC1 : Subsystem  mask(simucat_dac){deviceID=0, boxNum=Box 5 (Analog Board), channel1=on, channel2=off, channel3=off, channel4=off, channel5=off, channel6=off, channel7=off, channel8=off, channel9=off, channel10=off, channel11=off, channel12=off, channel13=off, channel14=off, channel15=off, channel16=off, channel17=off, channel18=off, channel19=off, channel20=off, calEnable=off, currentMode=off}
      mask prompts: deviceID "Device Index:"; boxNum "Select a box:"; channel1 "1"; channel2 "2"; channel3 "3"; channel4 "4"; channel5 "5"; channel6 "6"; channel7 "7"; channel8 "8"; channel9 "9"; channel10 "10"; channel11 "11"; channel12 "12"; channel13 "13"; channel14 "14"; channel15 "15"; channel16 "16"; channel17 "17"; channel18 "18"; channel19 "19"; channel20 "20"; calEnable "Enable DAC Calibrate"; currentMode "Apply Last 4 Channels(17~20) with Current Mode"
      mask help:
      | SimuCat系列模拟板卡驱动模块。
      | 功能：数字量转换模拟量。通道数：20
      settings: OpenFcn=open_system(gcb, 'mask');
      mask TypeOptions deviceID: 0 | 1 | 2 | 3 | 4 | 5 | 6 | 7 | 8 | 9 | 10 | 11 | 12 | 13 | 14 | 15
      mask TypeOptions boxNum: Box 5 (Analog Board) | Box 6 (Analog Board) | Box 7 (Analog Board)
      mask DialogControl refreshButton Prompt: Refresh
      mask DialogControl refreshButton Callback: ystbx.mask.callbacks.refreshBoxList
      mask DialogControl selectChannel Prompt: Select channels:
      mask DialogControl Dummy Prompt: (Add text here)
      mask DialogControl channelSelectAll Prompt: Select All
      mask DialogControl channelSelectAll Callback: ystbx.mask.callbacks.selectAllChannels();
      mask DialogControl channelClearAll Prompt: Clear All
      mask DialogControl channelClearAll Callback: ystbx.mask.callbacks.clearAllChannels();
      mask DialogControl applyButton Prompt: Apply Modification
      mask DialogControl applyButton Callback: ystbx.mask.callbacks.maskApply();
      mask Display: disp('CB2020(Analog Board)\ndigital-to-analog converter\nNetwork Device 0\nBox 5 (Analog Board)');port_label('input',1,'DAC_CH1[V]');
  DAC_CH1 : Constant  Commented=on  Value=0  OutDataTypeStr=double
  Gain1 : Gain
  Gain12 : Gain
  Gain2 : Gain
  Terminator1 : Terminator
  Terminator12 : Terminator
  Terminator2 : Terminator
  mean1 : Subsystem
  mean2 : Subsystem
  mean3 : Subsystem
  tag scope: Current_U=global, Current_V=global, Current_W=global
  wires:
  [Pressure_V] -> DAC1/1(DAC_CH1[V])  "DAC_CH1"
  AI3/1(Cur) -> [Current_W], Gain2/1  "ADC_CH3"
  AI2/1(Cur) -> [Current_V], Gain1/1  "ADC_CH2"
  AI1/1(Cur) -> [Current_U], Gain12/1  "ADC_CH1"
  mean1/1(Vol) -> AI1/1(Vol)
  mean2/1(Vol) -> AI2/1(Vol)
  mean3/1(Vol) -> AI3/1(Vol)
  Gain12/1 -> Terminator12/1
  Gain1/1 -> Terminator1/1
  Gain2/1 -> Terminator2/1
  ADC/1(ADC_CH1[V]) -> mean1/1(In1)
  ADC/2(ADC_CH2[V]) -> mean2/1(In1)
  ADC/3(ADC_CH3[V]) -> mean3/1(In1)

== system EHB_speedgoat_R2020a_V1/TIF_04/CB2020_2 ==
  ADC : Subsystem  mask(simucat_adc){deviceID=0, boxNum=Box 6 (Analog Board), channel1=on, channel2=on, channel3=on, channel4=on, channel5=on, channel6=on, channel7=on, channel8=on, channel9=on, channel10=on, channel11=on, channel12=on, channel13=on, channel14=on, channel15=on, channel16=on}
      mask prompts: deviceID "Device Index:"; boxNum "Select a box:"; channel1 "1"; channel2 "2"; channel3 "3"; channel4 "4"; channel5 "5"; channel6 "6"; channel7 "7"; channel8 "8"; channel9 "9"; channel10 "10"; channel11 "11"; channel12 "12"; channel13 "13"; channel14 "14"; channel15 "15"; channel16 "16"
      mask help:
      | SimuCat系列模拟板卡驱动模块。
      | 功能：模拟量转换数字量。通道数：16
      mask TypeOptions deviceID: 0 | 1 | 2 | 3 | 4 | 5 | 6 | 7 | 8 | 9 | 10 | 11 | 12 | 13 | 14 | 15
      mask TypeOptions boxNum: Box 5 (Analog Board) | Box 6 (Analog Board) | Box 7 (Analog Board)
      mask DialogControl refreshButton Prompt: Refresh
      mask DialogControl refreshButton Callback: ystbx.mask.callbacks.refreshBoxList
      mask DialogControl selectChannel Prompt: Select channels:
      mask DialogControl Dummy Prompt: (Add text here)
      mask DialogControl channelSelectAll Prompt: Select All
      mask DialogControl channelSelectAll Callback: ystbx.mask.callbacks.selectAllChannels();
      mask DialogControl channelClearAll Prompt: Clear All
      mask DialogControl channelClearAll Callback: ystbx.mask.callbacks.clearAllChannels();
      mask DialogControl applyButton Prompt: Apply Modification
      mask DialogControl applyButton Callback: ystbx.mask.callbacks.maskApply();
      mask Display: disp('CB2020(Analog Board)\nanalog-to-digital converter\nNetwork Device 0\nBox 6 (Analog Board)');port_label('output',1,'ADC_CH1[V]');port_label('output',2,'ADC_CH2[V]');port_label('output',3,'ADC_CH3[V]');port_label('output',4,'ADC_CH4[V]');port_label('output',5,'ADC_CH5[V]');port_label('output',6,'ADC_CH6[V]');port_label('output',7,'ADC_CH7[V]');port_label('output',8,'ADC_CH8[V]');port_label('output',9,'ADC_CH9[V]');port_label('output',10,'ADC_CH10[V]');port_label('output',11,'ADC_CH11[V]');port_label('output',12,'ADC_CH12[V]');port_label('output',13,'ADC_CH13[V]');port_label('output',14,'ADC_CH14[V]');port_label('output',15,'ADC_CH15[V]');port_label('output',16,'ADC_CH16[V]');
  AI1 : Subsystem
  AI10 : Subsystem
  AI11 : Subsystem
  AI12 : Subsystem
  AI13 : Subsystem
  AI14 : Subsystem
  AI15 : Subsystem
  AI16 : Subsystem
  AI2 : Subsystem
  AI3 : Subsystem
  AI4 : Subsystem
  AI5 : Subsystem
  AI6 : Subsystem
  AI7 : Subsystem
  AI8 : Subsystem
  AI9 : Subsystem
  DAC : Subsystem  mask(simucat_dac){deviceID=0, boxNum=Box 6 (Analog Board), channel1=on, channel2=on, channel3=on, channel4=on, channel5=on, channel6=on, channel7=on, channel8=on, channel9=on, channel10=on, channel11=on, channel12=on, channel13=on, channel14=on, channel15=on, channel16=on, channel17=on, channel18=on, channel19=on, channel20=on, calEnable=off}
      mask prompts: deviceID "Device Index:"; boxNum "Select a box:"; channel1 "1"; channel2 "2"; channel3 "3"; channel4 "4"; channel5 "5"; channel6 "6"; channel7 "7"; channel8 "8"; channel9 "9"; channel10 "10"; channel11 "11"; channel12 "12"; channel13 "13"; channel14 "14"; channel15 "15"; channel16 "16"; channel17 "17"; channel18 "18"; channel19 "19"; channel20 "20"; calEnable "Enable DAC Calibrate"
      mask help:
      | SimuCat系列模拟板卡驱动模块。
      | 功能：数字量转换模拟量。通道数：20
      mask TypeOptions deviceID: 0 | 1 | 2 | 3 | 4 | 5 | 6 | 7 | 8 | 9 | 10 | 11 | 12 | 13 | 14 | 15
      mask TypeOptions boxNum: Box 5 (Analog Board) | Box 6 (Analog Board) | Box 7 (Analog Board)
      mask DialogControl refreshButton Prompt: Refresh
      mask DialogControl refreshButton Callback: ystbx.mask.callbacks.refreshBoxList
      mask DialogControl selectChannel Prompt: Select channels:
      mask DialogControl Dummy Prompt: (Add text here)
      mask DialogControl channelSelectAll Prompt: Select All
      mask DialogControl channelSelectAll Callback: ystbx.mask.callbacks.selectAllChannels();
      mask DialogControl channelClearAll Prompt: Clear All
      mask DialogControl channelClearAll Callback: ystbx.mask.callbacks.clearAllChannels();
      mask DialogControl applyButton Prompt: Apply Modification
      mask DialogControl applyButton Callback: ystbx.mask.callbacks.maskApply();
      mask Display: disp('CB2020(Analog Board)\ndigital-to-analog converter\nNetwork Device 0\nBox 6 (Analog Board)');port_label('input',1,'DAC_CH1[V]');port_label('input',2,'DAC_CH2[V]');port_label('input',3,'DAC_CH3[V]');port_label('input',4,'DAC_CH4[V]');port_label('input',5,'DAC_CH5[V]');port_label('input',6,'DAC_CH6[V]');port_label('input',7,'DAC_CH7[V]');port_label('input',8,'DAC_CH8[V]');port_label('input',9,'DAC_CH9[V]');port_label('input',10,'DAC_CH10[V]');port_label('input',11,'DAC_CH11[V]');port_label('input',12,'DAC_CH12[V]');port_label('input',13,'DAC_CH13[V]');port_label('input',14,'DAC_CH14[V]');port_label('input',15,'DAC_CH15[V]');port_label('input',16,'DAC_CH16[V]');port_label('input',17,'DAC_CH17[V]');port_label('input',18,'DAC_CH18[V]');port_label('input',19,'DAC_CH19[V]');port_label('input',20,'DAC_CH20[V]');
  DAC_CH{1..11} (11 alike) : Constant  OutDataTypeStr=Inherit: Inherit via back propagation
  DAC_CH{12..20} (9 alike) : Constant  Value=0  OutDataTypeStr=Inherit: Inherit via back propagation
  Display{1..4,18..23,25..30} (16 alike) : Display
  mean1 : Subsystem
  mean10 : Subsystem
  mean11 : Subsystem
  mean12 : Subsystem
  mean13 : Subsystem
  mean14 : Subsystem
  mean15 : Subsystem
  mean16 : Subsystem
  mean2 : Subsystem
  mean3 : Subsystem
  mean4 : Subsystem
  mean5 : Subsystem
  mean6 : Subsystem
  mean7 : Subsystem
  mean8 : Subsystem
  mean9 : Subsystem
  wires:
  DAC_CH1/1 -> DAC/1(DAC_CH1[V])  "DAC_CH1"
  DAC_CH2/1 -> DAC/2(DAC_CH2[V])  "DAC_CH2"
  DAC_CH3/1 -> DAC/3(DAC_CH3[V])  "DAC_CH3"
  DAC_CH4/1 -> DAC/4(DAC_CH4[V])  "DAC_CH4"
  DAC_CH5/1 -> DAC/5(DAC_CH5[V])  "DAC_CH5"
  DAC_CH6/1 -> DAC/6(DAC_CH6[V])  "DAC_CH6"
  DAC_CH7/1 -> DAC/7(DAC_CH7[V])  "DAC_CH7"
  DAC_CH8/1 -> DAC/8(DAC_CH8[V])  "DAC_CH8"
  DAC_CH9/1 -> DAC/9(DAC_CH9[V])  "DAC_CH9"
  DAC_CH10/1 -> DAC/10(DAC_CH10[V])  "DAC_CH10"
  DAC_CH11/1 -> DAC/11(DAC_CH11[V])  "DAC_CH11"
  DAC_CH12/1 -> DAC/12(DAC_CH12[V])  "DAC_CH12"
  DAC_CH13/1 -> DAC/13(DAC_CH13[V])  "DAC_CH13"
  DAC_CH14/1 -> DAC/14(DAC_CH14[V])  "DAC_CH14"
  DAC_CH15/1 -> DAC/15(DAC_CH15[V])  "DAC_CH15"
  DAC_CH16/1 -> DAC/16(DAC_CH16[V])  "DAC_CH16"
  DAC_CH17/1 -> DAC/17(DAC_CH17[V])  "DAC_CH17"
  DAC_CH18/1 -> DAC/18(DAC_CH18[V])  "DAC_CH18"
  DAC_CH19/1 -> DAC/19(DAC_CH19[V])  "DAC_CH19"
  DAC_CH20/1 -> DAC/20(DAC_CH20[V])  "DAC_CH20"
  AI1/1(Cur) -> Display18/1  "ADC_CH21"
  AI13/1(Cur) -> Display30/1  "ADC_CH32"
  AI6/1(Cur) -> Display23/1  "ADC_CH26"
  AI2/1(Cur) -> Display19/1  "ADC_CH22"
  AI4/1(Cur) -> Display21/1  "ADC_CH24"
  AI8/1(Cur) -> Display25/1  "ADC_CH27"
  AI5/1(Cur) -> Display22/1  "ADC_CH25"
  AI3/1(Cur) -> Display20/1  "ADC_CH23"
  AI12/1(Cur) -> Display28/1  "ADC_CH31"
  AI10/1(Cur) -> Display29/1  "ADC_CH29"
  AI11/1(Cur) -> Display27/1  "ADC_CH30"
  AI9/1(Cur) -> Display26/1  "ADC_CH28"
  AI7/1(Cur) -> Display1/1  "ADC_CH27"
  AI16/1(Cur) -> Display4/1  "ADC_CH32"
  AI14/1(Cur) -> Display2/1  "ADC_CH30"
  AI15/1(Cur) -> Display3/1  "ADC_CH31"
  mean1/1(Vol) -> AI1/1(Vol)
  mean2/1(Vol) -> AI2/1(Vol)
  mean3/1(Vol) -> AI3/1(Vol)
  mean4/1(Vol) -> AI4/1(Vol)
  mean5/1(Vol) -> AI5/1(Vol)
  mean6/1(Vol) -> AI6/1(Vol)
  mean7/1(Vol) -> AI7/1(Vol)
  mean8/1(Vol) -> AI8/1(Vol)
  mean9/1(Vol) -> AI9/1(Vol)
  mean10/1(Vol) -> AI10/1(Vol)
  mean11/1(Vol) -> AI11/1(Vol)
  mean12/1(Vol) -> AI12/1(Vol)
  mean13/1(Vol) -> AI13/1(Vol)
  mean14/1(Vol) -> AI14/1(Vol)
  mean16/1(Vol) -> AI16/1(Vol)
  mean15/1(Vol) -> AI15/1(Vol)
  ADC/1(ADC_CH1[V]) -> mean1/1(In1)
  ADC/2(ADC_CH2[V]) -> mean2/1(In1)
  ADC/3(ADC_CH3[V]) -> mean3/1(In1)
  ADC/4(ADC_CH4[V]) -> mean4/1(In1)
  ADC/5(ADC_CH5[V]) -> mean5/1(In1)
  ADC/6(ADC_CH6[V]) -> mean6/1(In1)
  ADC/7(ADC_CH7[V]) -> mean7/1(In1)
  ADC/8(ADC_CH8[V]) -> mean8/1(In1)
  ADC/9(ADC_CH9[V]) -> mean9/1(In1)
  ADC/10(ADC_CH10[V]) -> mean10/1(In1)
  ADC/11(ADC_CH11[V]) -> mean11/1(In1)
  ADC/12(ADC_CH12[V]) -> mean12/1(In1)
  ADC/13(ADC_CH13[V]) -> mean13/1(In1)
  ADC/14(ADC_CH14[V]) -> mean14/1(In1)
  ADC/15(ADC_CH15[V]) -> mean15/1(In1)
  ADC/16(ADC_CH16[V]) -> mean16/1(In1)
